simulink model "ClosedLoop_System_Simulink"  (R2018a)
settings: Solver=ode4  StartTime=0.0  StopTime=t_final  FixedStep=dt  RelTol=1e-3
values from neighbouring files (symbols this model uses):
  e_IC = 20    [Nonlinear_Control_HW3_Q1_part_b.m]    (also in Nonlinear_Control_HW3_Q1_part_c.m; Nonlinear_Control_HW3_Q1_part_e.m = 64.66)
  K = 150    [Nonlinear_Control_HW3_Q1_part_a.m]    (also in Nonlinear_Control_HW3_Q1_part_b.m = 1; Nonlinear_Control_HW3_Q1_part_c.m = K_3(i); Nonlinear_Control_HW3_Q1_part_e.m)
settings Model: Creator=CF  LastModifiedBy=CF

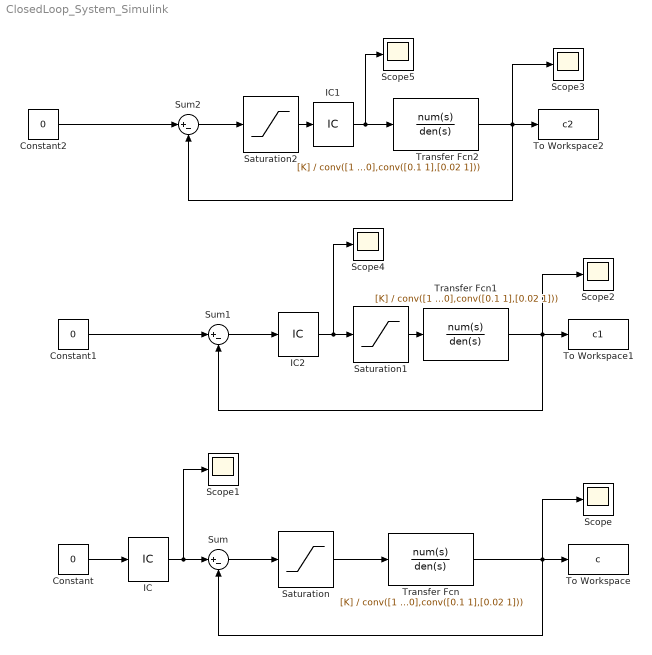
== system ClosedLoop_System_Simulink ==
  Constant : Constant  Value=0
  Constant1 : Constant  Value=0
  Constant2 : Constant  Value=0
  IC : InitialCondition  Value=e_IC
  IC1 : InitialCondition  Value=e_IC
  IC2 : InitialCondition  Value=e_IC
  Saturation : Saturate  UpperLimit=20  LowerLimit=-20
  Saturation1 : Saturate  UpperLimit=20  LowerLimit=-20
  Saturation2 : Saturate  UpperLimit=20  LowerLimit=-20
  Scope{,1..5} (6 alike) : Scope
  Sum : Sum  Inputs=|+-
  Sum1 : Sum  Inputs=|+-
  Sum2 : Sum  Inputs=|+-
  To Workspace : ToWorkspace  VariableName=c  SampleTime=-1
  To Workspace1 : ToWorkspace  VariableName=c1  SampleTime=-1
  To Workspace2 : ToWorkspace  VariableName=c2  SampleTime=-1
  Transfer Fcn : TransferFcn  Numerator=[K]  Denominator=conv([1 0],conv([0.1 1],[0.02 1]))
  Transfer Fcn1 : TransferFcn  Numerator=[K]  Denominator=conv([1 0],conv([0.1 1],[0.02 1]))
  Transfer Fcn2 : TransferFcn  Numerator=[K]  Denominator=conv([1 0],conv([0.1 1],[0.02 1]))
  wires:
  Saturation/1 -> Transfer Fcn/1
  Transfer Fcn/1 -> Scope/1, Sum/2, To Workspace/1
  Sum/1 -> Saturation/1
  IC/1 -> Scope1/1, Sum/1
  Constant/1 -> IC/1
  Constant1/1 -> Sum1/1
  Transfer Fcn1/1 -> Scope2/1, Sum1/2, To Workspace1/1
  Saturation1/1 -> Transfer Fcn1/1
  Sum1/1 -> IC2/1
  IC2/1 -> Scope4/1, Saturation1/1
  Constant2/1 -> Sum2/1
  Transfer Fcn2/1 -> Scope3/1, Sum2/2, To Workspace2/1
  Sum2/1 -> Saturation2/1
  IC1/1 -> Scope5/1, Transfer Fcn2/1
  Saturation2/1 -> IC1/1
